simulink model "MCov_AR"  (Simulink 7.1)
settings: Solver=FixedStepDiscrete  StartTime=0.0  StopTime=inf  RelTol=1e-3  AbsTol=1e-6
undefined symbols (not defined in the file or in its folder): bit, dfilt
libraries: c6713dsklib x2, dspspect3 x2, dsparch4 x1, etargetslib x1
settings Model: RequirementInfo=9  Creator=The MathWorks Inc.  LastModifiedBy=jfaing  ExtModeTrigMode=oneshot  ExtModeArmWhenConnect=off  ExtModeAutoUpdateStatusClock=off  BufferReuse=off
settings SolverCC: PositivePriorityOrder=on
settings DataIOCC: LimitDataPoints=off  SaveOutput=off  SaveTime=off  SignalLoggingName=sigsOut
settings OptimizationCC: BlockReduction=off  BooleanDataType=off  OptimizeBlockIOStorage=off  BufferReuse=off  ExpressionFolding=off  LocalBlockOutputs=off  RollThreshold=2  OptimizeModelRefInitCode=on  BufferReusableBoundary=off
settings DebuggingCC: SaveWithParameterizedLinksMsg=none  SignalResolutionControl=TryResolveAllWithWarning  SolverPrmCheckMsg=none  MultiTaskDSMMsg=warning  MultiTaskCondExecSysMsg=none  IntegerOverflowMsg=none  BusObjectLabelMismatch=none  StrictBusMsg=None
settings HardwareCC: ProdBitPerLong=40  ProdIntDivRoundTo=Zero  ProdEndianess=LittleEndian  ProdHWDeviceType=TI C6000  TargetHWDeviceType=32-bit Generic
settings RTWCC: SystemTargetFile=ti_c6000_ert.tlc  GenCodeOnly=on  TemplateMakefile=ti_c6000_ert.tmf  Description=Embedded Target for TI C6000 DSP (ERT)  ProcessScript=ti_c6000_ert_make_rtw_hook  IncludeERTFirstTime=on
settings CodeAppCC: IgnoreCustomStorageClasses=off
settings C6000ERTTargetCC: TargetFcnLib=ansi_tfl_tmw.mat  TargetFunctionLibrary=ANSI_C  UtilityFuncGeneration=Auto  GenerateFullHeader=on  GenerateSampleERTMain=off  GenerateTestInterfaces=off  IsPILTarget=off  ModelReferenceCompliant=on  CompOptLevelCompliant=off  IncludeMdlTerminateFcn=on  CombineOutputUpdateFcns=on  SuppressErrorStatus=off  ERTFirstTimeCompliant=off  IncludeFileDelimiter=Auto  ERTCustomFileBanners=on  SupportAbsoluteTime=on  LogVarNameModifier=rt_  MatFileLogging=off  MultiInstanceERTCode=off  SupportNonFinite=on  SupportComplex=on  PurelyIntegerCode=off  SupportContinuousTime=off  SupportNonInlinedSFcns=off  EnableShiftOperators=on  ParenthesesLevel=Nominal  PortableWordSizes=off  ModelStepFunctionPrototypeControlCompliant=off  AutosarCompliant=off  GenerateErtSFunction=off  GenerateASAP2=off  ExtMode=off  ExtModeTransport=0  ExtModeStaticAlloc=on  ExtModeStaticAllocSize=1000000  ExtModeTesting=off  ExtModeMexFile=noextcomm  ExtModeIntrfLevel=Level1  InlinedParameterPlacement=NonHierarchical  TargetOS=BareBoardExample  MultiInstanceErrorCode=Error  RateGroupingCode=on  RootIOFormat=Individual arguments  RTWCAPISignals=off  RTWCAPIParams=off  RTWCAPIStates=off  ERTSrcFileBannerTemplate=ert_code_template.cgt  ERTHdrFileBannerTemplate=ert_code_template.cgt  ERTDataSrcFileTemplate=ert_code_template.cgt  ERTDataHdrFileTemplate=ert_code_template.cgt  ERTCustomFileTemplate=example_file_process.tlc  ModuleNamingRule=Unspecified  SignalDisplayLevel=10  ParamTuneLevel=10  GlobalDataDefinition=Auto  DataDefinitionFile=global.c  GlobalDataReference=Auto  DataReferenceFile=global.h  GRTInterface=off  PreserveExpressionOrder=off  PreserveIfCondition=off  EnableUserReplacementTypes=off  MemSecPackage=--- None ---  MemSecDataConstants=Default  MemSecDataIO=Default  MemSecDataInternal=Default  MemSecDataParameters=Default  MemSecFuncInitTerm=Default  MemSecFuncExecute=Default  exportCCSObj=on  ccsObjName=CCS_Obj  useDSPBIOS=on  ProfileGenCode=off  InlineDSPBlks=on  FPopt=off  memModel=Far_Aggregate  optLevel=Function(-o2)  CompilerVerbosity=Quiet  InterruptThreshOnC6x=off  SymbolicDebugOnC6x=off  RetainAsmFiles=off  RetainObjFiles=on  CreateMapFile=on  UserStackSize=8192  c6000BuildAction=Build  OverrunAction=Notify_and_continue  OverrunNotificationMethod=Turn_on_LEDs

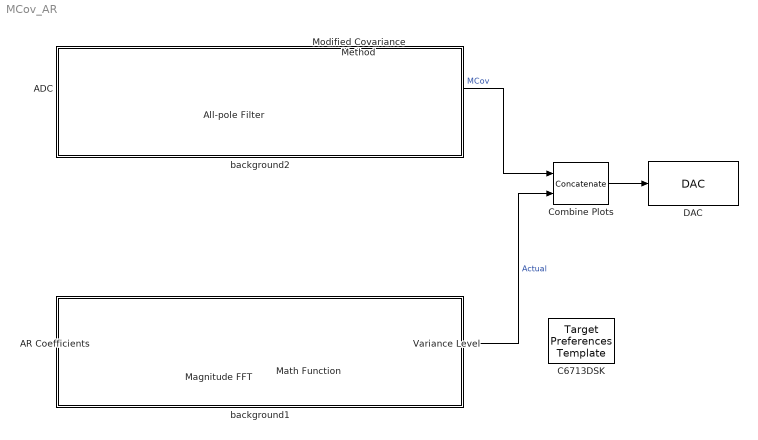
== system MCov_AR ==
  ADC : c6713dsklib/ADC  ADCsource=Line In  MicGain=off  Stereo=off  SampleRate=8 kHz  CodecDataFormat=16-bit  OutputDataType=Single  Scaling=Normalize  SourceGain=0.0  FrameSize=64  inheritSampleTime=off
  AR Coefficients : Constant  Value=[1 -2.2137 2.9403 -2.1697 0.9606]  OutDataTypeMode=single  OutDataType=sfix(16)  OutScaling=2^0  OutDataTypeStr=single
  All-pole Filter : dsparch4/Digital Filter  DialogController=dspdialog.DigitalFilter  DialogControllerArgs=DataTag0  TypePopup=IIR (all poles)  IIRFiltStruct=Direct form II transposed  AllPoleFiltStruct=Direct form  FIRFiltStruct=Direct form  CoeffSource=Specify via dialog  NumCoeffs=[1 2]  DenCoeffs=[1 -2.2137 2.9403 -2.1697 0.9606]  BiQuadCoeffs=[1 0.3 0.4 1 0.1 0.2]  LatticeCoeffs=[0.2 0.4]  denIgnore=on  FiltPerSampPopup=One filter per frame  IC=0  ICnum=0  ICden=0  roundingMode=Floor  overflowMode=off  ScaleValues=1  scaleValueFracLength=14  stageInFracLength=15  stageOutFracLength=15  FilterSource=Specify via dialog  dfiltObjectName=dfilt.dffir([1 2 1])
  C6713DSK : etargetslib/Target Preferences Template  Tag=C6000 TARGET PREFERENCES BLOCK  SystemSampleTime=-1
  Combine Plots : Concatenate  Mode=Multidimensional array  ConcatenateDimension=2
  DAC : c6713dsklib/DAC  CodecDataFormat=16-bit  SampleRate=8 kHz  Scaling=Normalize  DacAtten=0.0  OverflowMode=Wrap
  Magnitude FFT : dspspect3/Magnitude FFT  SystemSampleTime=-1  mag_or_magsq=Magnitude squared  fftLenInherit=off  fftsize=128
  Math Function : Math  Operator=reciprocal  OutDataType=sfix(16)  OutScaling=2^0  SaturateOnIntegerOverflow=on
  Modified Covariance Method : dspspect3/Modified Covariance Method  SystemSampleTime=-1  ord=4  inheritFFT=off  fftsize=128
  Variance Level : Gain  Gain=0.1  ParameterDataType=sfix(16)  ParameterScaling=2^0  OutDataType=sfix(16)  OutScaling=2^0  SaturateOnIntegerOverflow=on  OutDataTypeStr=Inherit: Same as input  ParamDataTypeStr=Inherit: Same as input
  background1 : Subsystem
      settings: AttributesFormatString=Actual Spectrum
      mask Display: disp('')
  background2 : Subsystem
      settings: AttributesFormatString=M-Cov Estimator
      mask Display: disp('')
  wires:
  Magnitude FFT/1 -> Math Function/1
  AR Coefficients/1 -> Magnitude FFT/1
  All-pole Filter/1 -> Modified Covariance Method/1
  Math Function/1 -> Variance Level/1
  Modified Covariance Method/1 -> Combine Plots/1  "MCov"
  Variance Level/1 -> Combine Plots/2  "Actual"
  Combine Plots/1 -> DAC/1
  ADC/1 -> All-pole Filter/1

== system MCov_AR/background1 ==

== system MCov_AR/background2 ==
